simulink model "AFO_sim1"  (R2020a)
settings: Solver=ode4  StartTime=0.0  StopTime=20  FixedStep=0.01  MaxStep=0.01  RelTol=1e-3  AbsTol=1e-3
PreLoadFcn:
  | addpath(genpath(pwd))
libraries: simulink x1
settings Model: Creator=12927  LastModifiedBy=12927
settings ModelReferenceCC: ModelReferenceMinAlgLoopOccurrences=on

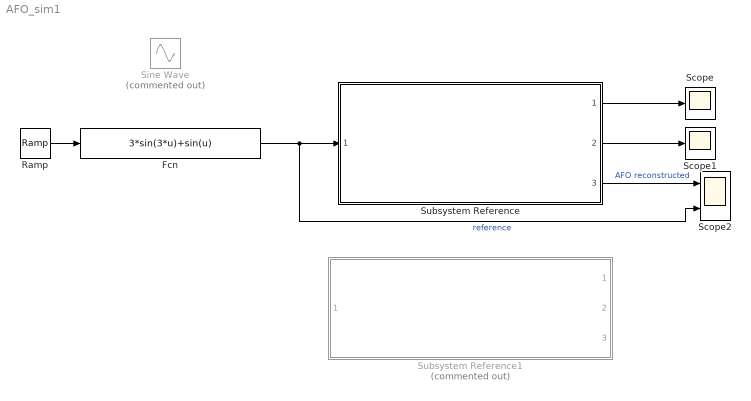
== system AFO_sim1 ==
  Fcn : Fcn  Expr=3*sin(3*u)+sin(u)
  Ramp : simulink/Sources/Ramp  slope=1  start=0  InitialOutput=0
  Scope : Scope
  Scope1 : Scope
  Scope2 : Scope  NumInputPorts=2
  Sine Wave : Sin  Commented=on  SampleTime=0
  Subsystem Reference : Subsystem  ReferencedSubsystem=AFO_network
  Subsystem Reference1 : Subsystem  Commented=on  ReferencedSubsystem=pDMP
  wires:
  Fcn/1 -> Scope2/2, Subsystem Reference/1  "reference"
  Subsystem Reference/1 -> Scope/1
  Subsystem Reference/2 -> Scope1/1
  Subsystem Reference/3 -> Scope2/1  "AFO reconstructed"
  Ramp/1 -> Fcn/1
